simulink model "Project5_trial"  (R2018b)
settings: Solver=VariableStepAuto  StartTime=0.0  StopTime=Sim_time  RelTol=1e-3
undefined symbols (not defined in the file or in its folder): Cn, I, OCV, R_Charge, R_Discharge, SOC
settings Model: Creator=Ismael  LastModifiedBy=Ismael

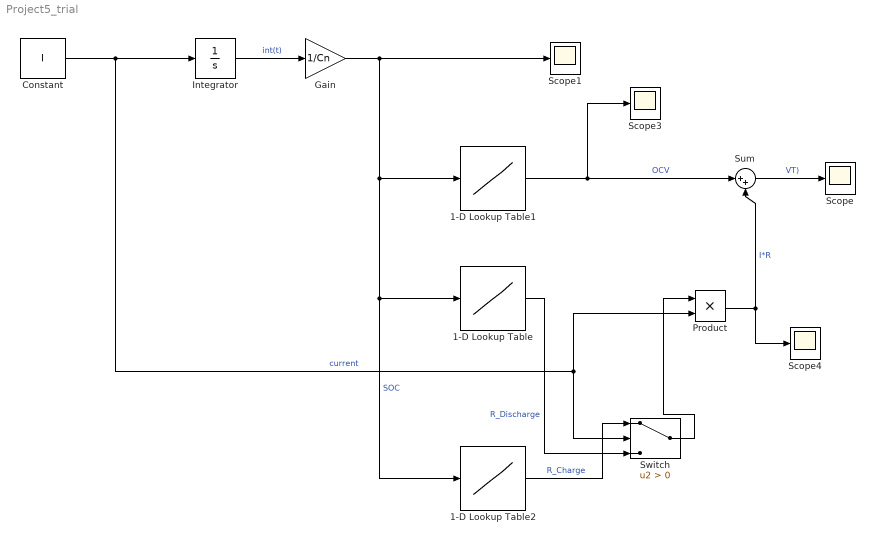
== system Project5_trial ==
  1-D Lookup Table : Lookup_n-D  NumberOfTableDimensions=1  BreakpointsForDimension1=SOC  Table=R_Discharge  InternalRulePriority=Speed  RndMeth=Simplest  InputSameDT=on
  1-D Lookup Table1 : Lookup_n-D  NumberOfTableDimensions=1  BreakpointsForDimension1=SOC  Table=OCV  InternalRulePriority=Speed  RndMeth=Simplest  InputSameDT=on
  1-D Lookup Table2 : Lookup_n-D  NumberOfTableDimensions=1  BreakpointsForDimension1=SOC  Table=R_Charge  InternalRulePriority=Speed  RndMeth=Simplest  InputSameDT=on
  Constant : Constant  Value=I
  Gain : Gain  Gain=1/Cn
  Integrator : Integrator
  Product : Product
  Scope{,1,3..4} (4 alike) : Scope
  Sum : Sum  Inputs=|++
  Switch : Switch  Criteria=u2 > Threshold
  wires:
  Constant/1 -> Switch/2, Product/2, Integrator/1  "current"
  Integrator/1 -> Gain/1  "int(t)"
  Gain/1 -> Scope1/1, 1-D Lookup Table2/1, 1-D Lookup Table/1, 1-D Lookup Table1/1  "SOC"
  1-D Lookup Table1/1 -> Scope3/1, Sum/1  "OCV"
  Product/1 -> Scope4/1, Sum/2  "I*R"
  Sum/1 -> Scope/1  "VT)"
  1-D Lookup Table/1 -> Switch/3  "R_Discharge"
  1-D Lookup Table2/1 -> Switch/1  "R_Charge"
  Switch/1 -> Product/1
